simulink model "lab2_model2"  (R2022a)
settings: Solver=VariableStepAuto  StartTime=0.0  StopTime=10.0  RelTol=1e-3
libraries: visiontextngfix x2
settings Model: Creator=User  LastModifiedBy=User

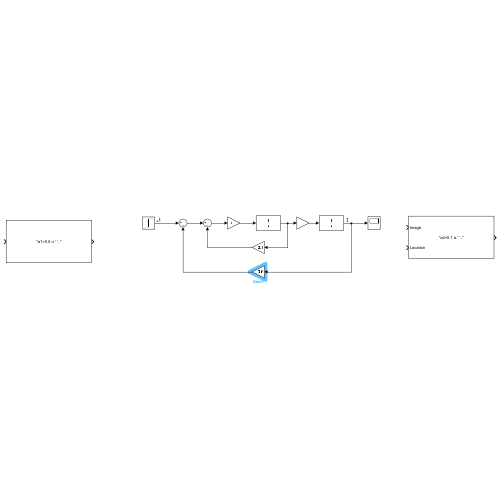
[thumbnail: Simulink's stored preview of the top-level diagram]
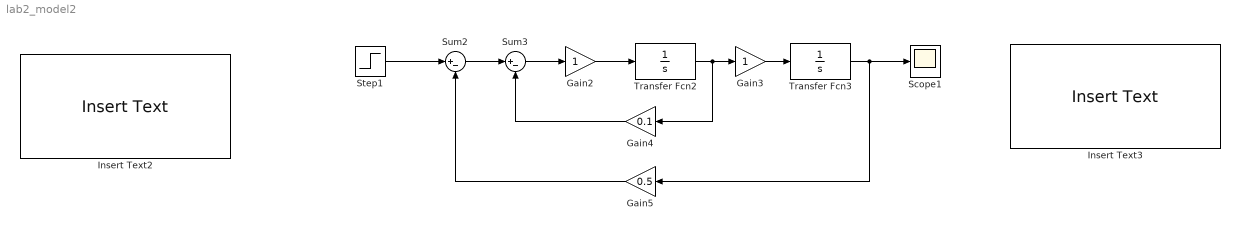
== system lab2_model2 ==
  Gain2 : Gain
  Gain3 : Gain
  Gain4 : Gain  Gain=0.1
  Gain5 : Gain  Gain=0.5
  Insert Text2 : visiontextngfix/Insert Text  inputType=Obsolete  theText='a1=0.5 периодический колебательный устойчивый a1=-0.5 периодический колебательный неустойчивый'  getTextLocFrom=Specify via dialog  textLoc=[1 1]  getTextColorFrom=Specify via dialog  textColor=[0 0 0]  getTextIntensityFrom=Specify via dialog  textIntensity=0  getTextOpacityFrom=Specify via dialog  textOpacity=1.0  dummyVar2=0  dummyVar3=0  dummyVar4=0  imagePorts=One multidimensional signal  isInputTransposed=off  fontFace=LucidaSansRegular  dummyVar1=0  blockFontSize=12  antiAliased=on
      settings: SourceProductBaseCode=VP
  Insert Text3 : visiontextngfix/Insert Text  inputType=Obsolete  theText='a2=0.1 апериодический устойчивый a2=0.8 апериодический устойчивый '  getTextLocFrom=Input port  textLoc=[1 1]  getTextColorFrom=Specify via dialog  textColor=[0 0 0]  getTextIntensityFrom=Specify via dialog  textIntensity=0  getTextOpacityFrom=Specify via dialog  textOpacity=1.0  dummyVar2=0  dummyVar3=0  dummyVar4=0  imagePorts=One multidimensional signal  isInputTransposed=off  fontFace=LucidaSansRegular  dummyVar1=0  blockFontSize=12  antiAliased=on
      settings: SourceProductBaseCode=VP
  Scope1 : Scope
  Step1 : Step  SampleTime=0
  Sum2 : Sum  Inputs=|+-
  Sum3 : Sum  Inputs=|+-
  Transfer Fcn2 : TransferFcn  Denominator=[1 0]
  Transfer Fcn3 : TransferFcn  Denominator=[1 0]
  wires:
  Transfer Fcn2/1 -> Gain4/1, Gain3/1
  Gain4/1 -> Sum3/2
  Step1/1 -> Sum2/1
  Gain5/1 -> Sum2/2
  Sum2/1 -> Sum3/1
  Sum3/1 -> Gain2/1
  Gain2/1 -> Transfer Fcn2/1
  Gain3/1 -> Transfer Fcn3/1
  Transfer Fcn3/1 -> Gain5/1, Scope1/1
